simulink model "quadrupedRobot"  (R2020a)
settings: Solver=ode23tb  StartTime=0.0  StopTime=10  RelTol=1e-3
values from neighbouring files (symbols this model uses):
  BodyCenter_To_Arm = BodyLength*0.4    (= 0.24)    [Initial.m]
  BodyLength = 0.6    [Initial.m]
  BodyThick = 0.05    [Initial.m]
  BodyWidth = 0.25    [Initial.m]
  L1 = 0.1*L_total    (= 0.05)    [Initial.m]
  L2 = 0.4*L_total    (= 0.2)    [Initial.m]
  L3 = 0.5*L_total    (= 0.25)    [Initial.m]
  L_total = 0.5    [Initial.m]
  legX = 0.05    [Initial.m]
  legY = 0.05    [Initial.m]
  legZ = 0.05    [Initial.m]
  Mark = 1    [Initial.m]
  X = R_foot*cosd(0:0.2:90)    [Initial.m]
  X_FOOT = ([x_swing x_stance])/1000-S/2/2/1000    [Initial.m]
  Y = R_foot*sind(0:0.2:90)    [Initial.m]
  Y_FOOT = L1    (= 0.05)    [Initial.m]
  Z_FOOT = -L2-L3+Z_trajectory/1000+0.15    [Initial.m]
undefined symbols (not defined in the file or in its folder): Z
libraries: sm_lib x84, nesl_utility x27, Contact_Forces_Lib x5, simulink x1
(part 4 of 4)

== system quadrupedRobot/Robot/RF/upperSys ==
  upperJoint : Inport
  PS-Simulink Converter : nesl_utility/PS-Simulink Converter  PhysicalDomain=network_engine_domain  SubClassName=ps_output  LeftPortType=input  RightPortType=output  PseudoPeriodic=off  Frequencies=[]  Unit=inherit  AffineConversion=off
  R2 : sm_lib/Joints/Revolute Joint  JointMode=Normal  SenseConstraintForce=off  SenseConstraintForceX=off  SenseConstraintForceY=off  SenseConstraintForceZ=off  SenseConstraintTorque=off  SenseConstraintTorqueX=off  SenseConstraintTorqueY=off  SenseConstraintTorqueZ=off  SenseTotalForce=off  SenseTotalForceX=off  SenseTotalForceY=off  SenseTotalForceZ=off  SenseTotalTorque=off  SenseTotalTorqueX=off  SenseTotalTorqueY=off  SenseTotalTorqueZ=off  CompositeWrenchDir=FollowerOnBase  CompositeWrenchFrame=BaseFrame  EquilibriumPosition=0  EquilibriumPositionUnits=deg  SpringStiffness=0  SpringStiffnessUnits=N*m/deg  DampingCoefficient=0  DampingCoefficientUnits=N*m/(deg/s)  TorqueActuationMode=ComputedTorque  MotionActuationMode=InputMotion  SensePosition=off  SenseVelocity=off  SenseAcceleration=off  SenseTorqueForce=on  SenseLowerLimitTorqueForce=off  SenseUpperLimitTorqueForce=off  LowerLimitSpecify=off  LowerLimitBound=-90  LowerLimitBoundUnits=deg  LowerLimitStiffness=1e4  LowerLimitStiffnessUnits=N*m/deg  LowerLimitDamping=10  LowerLimitDampingUnits=N*m/(deg/s)  LowerLimitTransitionRegionWidth=0.1  LowerLimitTransitionRegionWidthUnits=deg  UpperLimitSpecify=off  UpperLimitBound=90  UpperLimitBoundUnits=deg  UpperLimitStiffness=1e4  UpperLimitStiffnessUnits=N*m/deg  UpperLimitDamping=10  UpperLimitDampingUnits=N*m/(deg/s)  UpperLimitTransitionRegionWidth=0.1  UpperLimitTransitionRegionWidthUnits=deg  PositionTargetSpecify=on  PositionTargetPriority=High  PositionTargetValue=0  PositionTargetValueUnits=deg  VelocityTargetSpecify=off  VelocityTargetPriority=High  VelocityTargetValue=0  VelocityTargetValueUnits=deg/s
  Rigid Transform8 : sm_lib/Frames and Transforms/Rigid Transform  TranslationMethod=None  TranslationStandardOffset=0  TranslationLengthUnit=m  TranslationStandardAxis=+Z  TranslationCartesianOffset=[0 0 0]  TranslationROffset=0  TranslationROffsetUnits=m  TranslationZOffset=0  TranslationZOffsetUnits=m  TranslationThetaOffset=0  TranslationThetaOffsetUnits=deg  RotationMethod=StandardAxis  RotationAngleUnits=deg  RotationStandardAxis=+X  RotationAngle=90  RotationArbitraryAxis=[0 0 1]  FollAlignAxisA=+X  BaseAlignAxisA=+Y  FollAlignAxisB=+Y  BaseAlignAxisB=+Z  RotationSequenceAxes=FollowerAxes  RotationSequence=XYX  RotationSequenceAngles=[0 0 0]  RotationSequenceAnglesUnits=deg  RotationMatrix=[1 0 0; 0 1 0; 0 0 1]
  Rigid Transform9 : sm_lib/Frames and Transforms/Rigid Transform  TranslationMethod=None  TranslationStandardOffset=0  TranslationLengthUnit=m  TranslationStandardAxis=+Z  TranslationCartesianOffset=[0 0 0]  TranslationROffset=0  TranslationROffsetUnits=m  TranslationZOffset=0  TranslationZOffsetUnits=m  TranslationThetaOffset=0  TranslationThetaOffsetUnits=deg  RotationMethod=StandardAxis  RotationAngleUnits=deg  RotationStandardAxis=+X  RotationAngle=90  RotationArbitraryAxis=[0 0 1]  FollAlignAxisA=+X  BaseAlignAxisA=+Y  FollAlignAxisB=+Y  BaseAlignAxisB=+Z  RotationSequenceAxes=FollowerAxes  RotationSequence=XYX  RotationSequenceAngles=[0 0 0]  RotationSequenceAnglesUnits=deg  RotationMatrix=[1 0 0; 0 1 0; 0 0 1]
  Simulink-PS Converter4 : nesl_utility/Simulink-PS Converter  PhysicalDomain=network_engine_domain  SubClassName=ps_input  LeftPortType=input  RightPortType=output  PseudoPeriodic=off  Frequencies=[]  NoiseDistribution=none  NoiseParameters=[]  Unit=1  AffineConversion=off  FilteringAndDerivatives=filter  SimscapeFilterOrder=2  InputFilterTimeConstant=0.001  UdotUserProvided=0
  B1 : PMIOPort  Side=Left
  B2 : PMIOPort  Port=2  Side=Right
  Torque : Outport
  wires:
  upperJoint/1 -> Simulink-PS Converter4/1
  PS-Simulink Converter/1 -> Torque/1
  connections:
  Rigid Transform9/LConn1 -- B2/RConn1
  Rigid Transform8/LConn1 -- B1/RConn1
  R2/RConn1 -- Rigid Transform9/RConn1
  Rigid Transform8/RConn1 -- R2/LConn1
  Simulink-PS Converter4/RConn1 -- R2/LConn2
  PS-Simulink Converter/LConn1 -- R2/RConn2

== system quadrupedRobot/Robot/RR/Subsystem ==
  shoulderJoint : Inport
  R1 : sm_lib/Joints/Revolute Joint  JointMode=Normal  SenseConstraintForce=off  SenseConstraintForceX=off  SenseConstraintForceY=off  SenseConstraintForceZ=off  SenseConstraintTorque=off  SenseConstraintTorqueX=off  SenseConstraintTorqueY=off  SenseConstraintTorqueZ=off  SenseTotalForce=off  SenseTotalForceX=off  SenseTotalForceY=off  SenseTotalForceZ=off  SenseTotalTorque=off  SenseTotalTorqueX=off  SenseTotalTorqueY=off  SenseTotalTorqueZ=off  CompositeWrenchDir=FollowerOnBase  CompositeWrenchFrame=BaseFrame  EquilibriumPosition=0  EquilibriumPositionUnits=deg  SpringStiffness=0  SpringStiffnessUnits=N*m/deg  DampingCoefficient=0  DampingCoefficientUnits=N*m/(deg/s)  TorqueActuationMode=ComputedTorque  MotionActuationMode=InputMotion  SensePosition=off  SenseVelocity=off  SenseAcceleration=off  SenseTorqueForce=off  SenseLowerLimitTorqueForce=off  SenseUpperLimitTorqueForce=off  LowerLimitSpecify=off  LowerLimitBound=-90  LowerLimitBoundUnits=deg  LowerLimitStiffness=1e4  LowerLimitStiffnessUnits=N*m/deg  LowerLimitDamping=10  LowerLimitDampingUnits=N*m/(deg/s)  LowerLimitTransitionRegionWidth=0.1  LowerLimitTransitionRegionWidthUnits=deg  UpperLimitSpecify=off  UpperLimitBound=90  UpperLimitBoundUnits=deg  UpperLimitStiffness=1e4  UpperLimitStiffnessUnits=N*m/deg  UpperLimitDamping=10  UpperLimitDampingUnits=N*m/(deg/s)  UpperLimitTransitionRegionWidth=0.1  UpperLimitTransitionRegionWidthUnits=deg  PositionTargetSpecify=on  PositionTargetPriority=High  PositionTargetValue=0  PositionTargetValueUnits=deg  VelocityTargetSpecify=off  VelocityTargetPriority=High  VelocityTargetValue=0  VelocityTargetValueUnits=deg/s
  Rigid Transform8 : sm_lib/Frames and Transforms/Rigid Transform  TranslationMethod=None  TranslationStandardOffset=0  TranslationLengthUnit=m  TranslationStandardAxis=+Z  TranslationCartesianOffset=[0 0 0]  TranslationROffset=0  TranslationROffsetUnits=m  TranslationZOffset=0  TranslationZOffsetUnits=m  TranslationThetaOffset=0  TranslationThetaOffsetUnits=deg  RotationMethod=StandardAxis  RotationAngleUnits=deg  RotationStandardAxis=+Y  RotationAngle=90  RotationArbitraryAxis=[0 0 1]  FollAlignAxisA=+X  BaseAlignAxisA=+Y  FollAlignAxisB=+Y  BaseAlignAxisB=+Z  RotationSequenceAxes=FollowerAxes  RotationSequence=XYX  RotationSequenceAngles=[0 0 0]  RotationSequenceAnglesUnits=deg  RotationMatrix=[1 0 0; 0 1 0; 0 0 1]
  Rigid Transform9 : sm_lib/Frames and Transforms/Rigid Transform  TranslationMethod=None  TranslationStandardOffset=0  TranslationLengthUnit=m  TranslationStandardAxis=+Z  TranslationCartesianOffset=[0 0 0]  TranslationROffset=0  TranslationROffsetUnits=m  TranslationZOffset=0  TranslationZOffsetUnits=m  TranslationThetaOffset=0  TranslationThetaOffsetUnits=deg  RotationMethod=StandardAxis  RotationAngleUnits=deg  RotationStandardAxis=+Y  RotationAngle=90  RotationArbitraryAxis=[0 0 1]  FollAlignAxisA=+X  BaseAlignAxisA=+Y  FollAlignAxisB=+Y  BaseAlignAxisB=+Z  RotationSequenceAxes=FollowerAxes  RotationSequence=XYX  RotationSequenceAngles=[0 0 0]  RotationSequenceAnglesUnits=deg  RotationMatrix=[1 0 0; 0 1 0; 0 0 1]
  Simulink-PS Converter4 : nesl_utility/Simulink-PS Converter  PhysicalDomain=network_engine_domain  SubClassName=ps_input  LeftPortType=input  RightPortType=output  PseudoPeriodic=off  Frequencies=[]  NoiseDistribution=none  NoiseParameters=[]  Unit=1  AffineConversion=off  FilteringAndDerivatives=filter  SimscapeFilterOrder=2  InputFilterTimeConstant=0.001  UdotUserProvided=0
  B1 : PMIOPort  Side=Left
  B2 : PMIOPort  Port=2  Side=Right
  wires:
  shoulderJoint/1 -> Simulink-PS Converter4/1
  connections:
  Rigid Transform8/RConn1 -- R1/LConn1
  Simulink-PS Converter4/RConn1 -- R1/LConn2
  R1/RConn1 -- Rigid Transform9/RConn1
  Rigid Transform8/LConn1 -- B1/RConn1
  Rigid Transform9/LConn1 -- B2/RConn1

== system quadrupedRobot/Robot/RR/Subsystem1 ==
  upperJoint : Inport
  R2 : sm_lib/Joints/Revolute Joint  JointMode=Normal  SenseConstraintForce=off  SenseConstraintForceX=off  SenseConstraintForceY=off  SenseConstraintForceZ=off  SenseConstraintTorque=off  SenseConstraintTorqueX=off  SenseConstraintTorqueY=off  SenseConstraintTorqueZ=off  SenseTotalForce=off  SenseTotalForceX=off  SenseTotalForceY=off  SenseTotalForceZ=off  SenseTotalTorque=off  SenseTotalTorqueX=off  SenseTotalTorqueY=off  SenseTotalTorqueZ=off  CompositeWrenchDir=FollowerOnBase  CompositeWrenchFrame=BaseFrame  EquilibriumPosition=0  EquilibriumPositionUnits=deg  SpringStiffness=0  SpringStiffnessUnits=N*m/deg  DampingCoefficient=0  DampingCoefficientUnits=N*m/(deg/s)  TorqueActuationMode=ComputedTorque  MotionActuationMode=InputMotion  SensePosition=off  SenseVelocity=off  SenseAcceleration=off  SenseTorqueForce=off  SenseLowerLimitTorqueForce=off  SenseUpperLimitTorqueForce=off  LowerLimitSpecify=off  LowerLimitBound=-90  LowerLimitBoundUnits=deg  LowerLimitStiffness=1e4  LowerLimitStiffnessUnits=N*m/deg  LowerLimitDamping=10  LowerLimitDampingUnits=N*m/(deg/s)  LowerLimitTransitionRegionWidth=0.1  LowerLimitTransitionRegionWidthUnits=deg  UpperLimitSpecify=off  UpperLimitBound=90  UpperLimitBoundUnits=deg  UpperLimitStiffness=1e4  UpperLimitStiffnessUnits=N*m/deg  UpperLimitDamping=10  UpperLimitDampingUnits=N*m/(deg/s)  UpperLimitTransitionRegionWidth=0.1  UpperLimitTransitionRegionWidthUnits=deg  PositionTargetSpecify=on  PositionTargetPriority=High  PositionTargetValue=0  PositionTargetValueUnits=deg  VelocityTargetSpecify=off  VelocityTargetPriority=High  VelocityTargetValue=0  VelocityTargetValueUnits=deg/s
  Rigid Transform8 : sm_lib/Frames and Transforms/Rigid Transform  TranslationMethod=None  TranslationStandardOffset=0  TranslationLengthUnit=m  TranslationStandardAxis=+Z  TranslationCartesianOffset=[0 0 0]  TranslationROffset=0  TranslationROffsetUnits=m  TranslationZOffset=0  TranslationZOffsetUnits=m  TranslationThetaOffset=0  TranslationThetaOffsetUnits=deg  RotationMethod=StandardAxis  RotationAngleUnits=deg  RotationStandardAxis=+X  RotationAngle=90  RotationArbitraryAxis=[0 0 1]  FollAlignAxisA=+X  BaseAlignAxisA=+Y  FollAlignAxisB=+Y  BaseAlignAxisB=+Z  RotationSequenceAxes=FollowerAxes  RotationSequence=XYX  RotationSequenceAngles=[0 0 0]  RotationSequenceAnglesUnits=deg  RotationMatrix=[1 0 0; 0 1 0; 0 0 1]
  Rigid Transform9 : sm_lib/Frames and Transforms/Rigid Transform  TranslationMethod=None  TranslationStandardOffset=0  TranslationLengthUnit=m  TranslationStandardAxis=+Z  TranslationCartesianOffset=[0 0 0]  TranslationROffset=0  TranslationROffsetUnits=m  TranslationZOffset=0  TranslationZOffsetUnits=m  TranslationThetaOffset=0  TranslationThetaOffsetUnits=deg  RotationMethod=StandardAxis  RotationAngleUnits=deg  RotationStandardAxis=+X  RotationAngle=90  RotationArbitraryAxis=[0 0 1]  FollAlignAxisA=+X  BaseAlignAxisA=+Y  FollAlignAxisB=+Y  BaseAlignAxisB=+Z  RotationSequenceAxes=FollowerAxes  RotationSequence=XYX  RotationSequenceAngles=[0 0 0]  RotationSequenceAnglesUnits=deg  RotationMatrix=[1 0 0; 0 1 0; 0 0 1]
  Simulink-PS Converter4 : nesl_utility/Simulink-PS Converter  PhysicalDomain=network_engine_domain  SubClassName=ps_input  LeftPortType=input  RightPortType=output  PseudoPeriodic=off  Frequencies=[]  NoiseDistribution=none  NoiseParameters=[]  Unit=1  AffineConversion=off  FilteringAndDerivatives=filter  SimscapeFilterOrder=2  InputFilterTimeConstant=0.001  UdotUserProvided=0
  B1 : PMIOPort  Side=Left
  B2 : PMIOPort  Port=2  Side=Right
  wires:
  upperJoint/1 -> Simulink-PS Converter4/1
  connections:
  Rigid Transform9/LConn1 -- B2/RConn1
  Rigid Transform8/LConn1 -- B1/RConn1
  R2/RConn1 -- Rigid Transform9/RConn1
  Rigid Transform8/RConn1 -- R2/LConn1
  Simulink-PS Converter4/RConn1 -- R2/LConn2

== system quadrupedRobot/Robot/RR/Subsystem2 ==
  lowerJoint : Inport
  R3 : sm_lib/Joints/Revolute Joint  JointMode=Normal  SenseConstraintForce=off  SenseConstraintForceX=off  SenseConstraintForceY=off  SenseConstraintForceZ=off  SenseConstraintTorque=off  SenseConstraintTorqueX=off  SenseConstraintTorqueY=off  SenseConstraintTorqueZ=off  SenseTotalForce=off  SenseTotalForceX=off  SenseTotalForceY=off  SenseTotalForceZ=off  SenseTotalTorque=off  SenseTotalTorqueX=off  SenseTotalTorqueY=off  SenseTotalTorqueZ=off  CompositeWrenchDir=FollowerOnBase  CompositeWrenchFrame=BaseFrame  EquilibriumPosition=0  EquilibriumPositionUnits=deg  SpringStiffness=0  SpringStiffnessUnits=N*m/deg  DampingCoefficient=0  DampingCoefficientUnits=N*m/(deg/s)  TorqueActuationMode=ComputedTorque  MotionActuationMode=InputMotion  SensePosition=off  SenseVelocity=off  SenseAcceleration=off  SenseTorqueForce=off  SenseLowerLimitTorqueForce=off  SenseUpperLimitTorqueForce=off  LowerLimitSpecify=off  LowerLimitBound=-90  LowerLimitBoundUnits=deg  LowerLimitStiffness=1e4  LowerLimitStiffnessUnits=N*m/deg  LowerLimitDamping=10  LowerLimitDampingUnits=N*m/(deg/s)  LowerLimitTransitionRegionWidth=0.1  LowerLimitTransitionRegionWidthUnits=deg  UpperLimitSpecify=off  UpperLimitBound=90  UpperLimitBoundUnits=deg  UpperLimitStiffness=1e4  UpperLimitStiffnessUnits=N*m/deg  UpperLimitDamping=10  UpperLimitDampingUnits=N*m/(deg/s)  UpperLimitTransitionRegionWidth=0.1  UpperLimitTransitionRegionWidthUnits=deg  PositionTargetSpecify=on  PositionTargetPriority=High  PositionTargetValue=0  PositionTargetValueUnits=deg  VelocityTargetSpecify=off  VelocityTargetPriority=High  VelocityTargetValue=0  VelocityTargetValueUnits=deg/s
  Rigid Transform8 : sm_lib/Frames and Transforms/Rigid Transform  TranslationMethod=None  TranslationStandardOffset=0  TranslationLengthUnit=m  TranslationStandardAxis=+Z  TranslationCartesianOffset=[0 0 0]  TranslationROffset=0  TranslationROffsetUnits=m  TranslationZOffset=0  TranslationZOffsetUnits=m  TranslationThetaOffset=0  TranslationThetaOffsetUnits=deg  RotationMethod=StandardAxis  RotationAngleUnits=deg  RotationStandardAxis=+X  RotationAngle=90  RotationArbitraryAxis=[0 0 1]  FollAlignAxisA=+X  BaseAlignAxisA=+Y  FollAlignAxisB=+Y  BaseAlignAxisB=+Z  RotationSequenceAxes=FollowerAxes  RotationSequence=XYX  RotationSequenceAngles=[0 0 0]  RotationSequenceAnglesUnits=deg  RotationMatrix=[1 0 0; 0 1 0; 0 0 1]
  Rigid Transform9 : sm_lib/Frames and Transforms/Rigid Transform  TranslationMethod=None  TranslationStandardOffset=0  TranslationLengthUnit=m  TranslationStandardAxis=+Z  TranslationCartesianOffset=[0 0 0]  TranslationROffset=0  TranslationROffsetUnits=m  TranslationZOffset=0  TranslationZOffsetUnits=m  TranslationThetaOffset=0  TranslationThetaOffsetUnits=deg  RotationMethod=StandardAxis  RotationAngleUnits=deg  RotationStandardAxis=+X  RotationAngle=90  RotationArbitraryAxis=[0 0 1]  FollAlignAxisA=+X  BaseAlignAxisA=+Y  FollAlignAxisB=+Y  BaseAlignAxisB=+Z  RotationSequenceAxes=FollowerAxes  RotationSequence=XYX  RotationSequenceAngles=[0 0 0]  RotationSequenceAnglesUnits=deg  RotationMatrix=[1 0 0; 0 1 0; 0 0 1]
  Simulink-PS Converter : nesl_utility/Simulink-PS Converter  PhysicalDomain=network_engine_domain  SubClassName=ps_input  LeftPortType=input  RightPortType=output  PseudoPeriodic=off  Frequencies=[]  NoiseDistribution=none  NoiseParameters=[]  Unit=1  AffineConversion=off  FilteringAndDerivatives=filter  SimscapeFilterOrder=2  InputFilterTimeConstant=0.001  UdotUserProvided=0
  B1 : PMIOPort  Side=Left
  B2 : PMIOPort  Port=2  Side=Right
  wires:
  lowerJoint/1 -> Simulink-PS Converter/1
  connections:
  Rigid Transform9/LConn1 -- B2/RConn1
  Rigid Transform8/LConn1 -- B1/RConn1
  R3/RConn1 -- Rigid Transform9/RConn1
  Simulink-PS Converter/RConn1 -- R3/LConn2
  Rigid Transform8/RConn1 -- R3/LConn1

== system quadrupedRobot/controller/原地机身ROLL PITCH YAW三角变化演示（正确）/LF_CONTROL ==
  Theta123 : Inport
  Demux : Demux  Outputs=3
  Gain : Gain  Gain=-1
  ToRad : Gain  Gain=pi/180
  tag scope: LF_lower=global, LF_shoulder=global, LF_upper=global
  wires:
  Theta123/1 -> ToRad/1
  Demux/3 -> [LF_lower]
  Demux/1 -> Gain/1
  Demux/2 -> [LF_upper]
  ToRad/1 -> Demux/1
  Gain/1 -> [LF_shoulder]

== system quadrupedRobot/controller/原地机身ROLL PITCH YAW三角变化演示（正确）/LR_CONTROL ==
  Theta123 : Inport
  Demux : Demux  Outputs=3
  Gain : Gain  Gain=-1
  ToRad : Gain  Gain=pi/180
  tag scope: LR_lower=global, LR_shoulder=global, LR_upper=global
  wires:
  Theta123/1 -> ToRad/1
  Demux/3 -> [LR_lower]
  Demux/1 -> Gain/1
  Demux/2 -> [LR_upper]
  ToRad/1 -> Demux/1
  Gain/1 -> [LR_shoulder]

== system quadrupedRobot/controller/原地机身ROLL PITCH YAW三角变化演示（正确）/RF_CONTROL ==
  Theta123 : Inport
  Demux : Demux  Outputs=3
  ToRad : Gain  Gain=pi/180
  tag scope: RF_lower=global, RF_shoulder=global, RF_upper=global
  wires:
  Demux/1 -> [RF_shoulder]
  Demux/3 -> [RF_lower]
  Demux/2 -> [RF_upper]
  Theta123/1 -> ToRad/1
  ToRad/1 -> Demux/1

== system quadrupedRobot/controller/原地机身ROLL PITCH YAW三角变化演示（正确）/RR_CONTROL ==
  Theta123 : Inport
  Demux : Demux  Outputs=3
  ToRad : Gain  Gain=pi/180
  tag scope: RR_lower=global, RR_shoulder=global, RR_upper=global
  wires:
  Theta123/1 -> ToRad/1
  Demux/3 -> [RR_lower]
  Demux/1 -> [RR_shoulder]
  Demux/2 -> [RR_upper]
  ToRad/1 -> Demux/1

== system quadrupedRobot/controller/原地机身ROLL PITCH YAW三角变化演示（正确）/初始位置发生器（每条腿相同） ==
  Init_X : Constant  Value=X_FOOT(1)
  Init_Y : Constant  Value=Y_FOOT(1)
  Init_Z : Constant  Value=Z_FOOT(1)
  Init_x : Outport
  Init_y : Outport  Port=2
  Init_z : Outport  Port=3
  wires:
  Init_X/1 -> Init_x/1
  Init_Y/1 -> Init_y/1
  Init_Z/1 -> Init_z/1

== system quadrupedRobot/controller/原地机身ROLL角变化演示/LF_CONTROL ==
  Theta123 : Inport
  Demux : Demux  Outputs=3
  Gain : Gain  Gain=-1
  ToRad : Gain  Gain=pi/180
  tag scope: LF_lower=global, LF_shoulder=global, LF_upper=global
  wires:
  Theta123/1 -> ToRad/1
  Demux/3 -> [LF_lower]
  Demux/1 -> Gain/1
  Demux/2 -> [LF_upper]
  ToRad/1 -> Demux/1
  Gain/1 -> [LF_shoulder]

== system quadrupedRobot/controller/原地机身ROLL角变化演示/LR_CONTROL ==
  Theta123 : Inport
  Demux : Demux  Outputs=3
  Gain : Gain  Gain=-1
  ToRad : Gain  Gain=pi/180
  tag scope: LR_lower=global, LR_shoulder=global, LR_upper=global
  wires:
  Theta123/1 -> ToRad/1
  Demux/3 -> [LR_lower]
  Demux/1 -> Gain/1
  Demux/2 -> [LR_upper]
  ToRad/1 -> Demux/1
  Gain/1 -> [LR_shoulder]

== system quadrupedRobot/controller/原地机身ROLL角变化演示/RF_CONTROL ==
  Theta123 : Inport
  Demux : Demux  Outputs=3
  ToRad : Gain  Gain=pi/180
  tag scope: RF_lower=global, RF_shoulder=global, RF_upper=global
  wires:
  Demux/1 -> [RF_shoulder]
  Demux/3 -> [RF_lower]
  Demux/2 -> [RF_upper]
  Theta123/1 -> ToRad/1
  ToRad/1 -> Demux/1

== system quadrupedRobot/controller/原地机身ROLL角变化演示/RR_CONTROL ==
  Theta123 : Inport
  Demux : Demux  Outputs=3
  ToRad : Gain  Gain=pi/180
  tag scope: RR_lower=global, RR_shoulder=global, RR_upper=global
  wires:
  Theta123/1 -> ToRad/1
  Demux/3 -> [RR_lower]
  Demux/1 -> [RR_shoulder]
  Demux/2 -> [RR_upper]
  ToRad/1 -> Demux/1

== system quadrupedRobot/controller/原地机身ROLL角变化演示/初始位置发生器（每条腿相同） ==
  Init_X : Constant  Value=X_FOOT(1)
  Init_Y : Constant  Value=L1
  Init_Z : Constant  Value=Z_FOOT(1)
  Init_x : Outport
  Init_y : Outport  Port=2
  Init_z : Outport  Port=3
  wires:
  Init_X/1 -> Init_x/1
  Init_Y/1 -> Init_y/1
  Init_Z/1 -> Init_z/1

== system quadrupedRobot/controller/原地机身YAW角变化演示（有误）/LF_CONTROL ==
  Theta123 : Inport
  Demux : Demux  Outputs=3
  Gain : Gain  Gain=-1
  ToRad : Gain  Gain=pi/180
  tag scope: LF_lower=global, LF_shoulder=global, LF_upper=global
  wires:
  Gain/1 -> [LF_shoulder]
  ToRad/1 -> Demux/1
  Demux/2 -> [LF_upper]
  Demux/1 -> Gain/1
  Demux/3 -> [LF_lower]
  Theta123/1 -> ToRad/1

== system quadrupedRobot/controller/原地机身YAW角变化演示（有误）/LR_CONTROL ==
  Theta123 : Inport
  Demux : Demux  Outputs=3
  Gain : Gain  Gain=-1
  ToRad : Gain  Gain=pi/180
  tag scope: LR_lower=global, LR_shoulder=global, LR_upper=global
  wires:
  Gain/1 -> [LR_shoulder]
  ToRad/1 -> Demux/1
  Demux/2 -> [LR_upper]
  Demux/1 -> Gain/1
  Demux/3 -> [LR_lower]
  Theta123/1 -> ToRad/1

== system quadrupedRobot/controller/原地机身YAW角变化演示（有误）/RF_CONTROL ==
  Theta123 : Inport
  Demux : Demux  Outputs=3
  ToRad : Gain  Gain=pi/180
  tag scope: RF_lower=global, RF_shoulder=global, RF_upper=global
  wires:
  ToRad/1 -> Demux/1
  Theta123/1 -> ToRad/1
  Demux/2 -> [RF_upper]
  Demux/3 -> [RF_lower]
  Demux/1 -> [RF_shoulder]

== system quadrupedRobot/controller/原地机身YAW角变化演示（有误）/RR_CONTROL ==
  Theta123 : Inport
  Demux : Demux  Outputs=3
  ToRad : Gain  Gain=pi/180
  tag scope: RR_lower=global, RR_shoulder=global, RR_upper=global
  wires:
  ToRad/1 -> Demux/1
  Demux/2 -> [RR_upper]
  Demux/1 -> [RR_shoulder]
  Demux/3 -> [RR_lower]
  Theta123/1 -> ToRad/1

== system quadrupedRobot/controller/原地机身YAW角变化演示（有误）/初始位置发生器（每条腿相同） ==
  Init_X : Constant  Value=X_FOOT(1)
  Init_Y : Constant  Value=Y_FOOT(1)
  Init_Z : Constant  Value=Z_FOOT(1)
  Init_x : Outport
  Init_y : Outport  Port=2
  Init_z : Outport  Port=3
  wires:
  Init_Z/1 -> Init_z/1
  Init_Y/1 -> Init_y/1
  Init_X/1 -> Init_x/1

== system quadrupedRobot/controller/对角步态演示/LF_CONTROL ==
  Theta123 : Inport
  Demux : Demux  Outputs=3
  Gain : Gain  Gain=-1
  ToRad : Gain  Gain=pi/180
  tag scope: LF_lower=global, LF_shoulder=global, LF_upper=global
  wires:
  Theta123/1 -> ToRad/1
  Demux/3 -> [LF_lower]
  Demux/1 -> Gain/1
  Demux/2 -> [LF_upper]
  ToRad/1 -> Demux/1
  Gain/1 -> [LF_shoulder]

== system quadrupedRobot/controller/对角步态演示/LR_CONTROL ==
  Theta123 : Inport
  Demux : Demux  Outputs=3
  Gain : Gain  Gain=-1
  ToRad : Gain  Gain=pi/180
  tag scope: LR_lower=global, LR_shoulder=global, LR_upper=global
  wires:
  Theta123/1 -> ToRad/1
  Demux/3 -> [LR_lower]
  Demux/1 -> Gain/1
  Demux/2 -> [LR_upper]
  ToRad/1 -> Demux/1
  Gain/1 -> [LR_shoulder]

== system quadrupedRobot/controller/对角步态演示/RF_CONTROL ==
  Theta123 : Inport
  Demux : Demux  Outputs=3
  ToRad : Gain  Gain=pi/180
  tag scope: RF_lower=global, RF_shoulder=global, RF_upper=global
  wires:
  Demux/1 -> [RF_shoulder]
  Demux/3 -> [RF_lower]
  Demux/2 -> [RF_upper]
  Theta123/1 -> ToRad/1
  ToRad/1 -> Demux/1

== system quadrupedRobot/controller/对角步态演示/RR_CONTROL ==
  Theta123 : Inport
  Demux : Demux  Outputs=3
  ToRad : Gain  Gain=pi/180
  tag scope: RR_lower=global, RR_shoulder=global, RR_upper=global
  wires:
  Theta123/1 -> ToRad/1
  Demux/3 -> [RR_lower]
  Demux/1 -> [RR_shoulder]
  Demux/2 -> [RR_upper]
  ToRad/1 -> Demux/1

== system quadrupedRobot/controller/对角步态演示/初始位置发生器（每条腿相同） ==
  Init_X : Constant  Value=X_FOOT(1)
  Init_Y : Constant  Value=Y_FOOT(1)
  Init_Z : Constant  Value=Z_FOOT(1)
  Init_x : Outport
  Init_y : Outport  Port=2
  Init_z : Outport  Port=3
  wires:
  Init_X/1 -> Init_x/1
  Init_Y/1 -> Init_y/1
  Init_Z/1 -> Init_z/1

== system quadrupedRobot/controller/对角步态演示/对角步态坐标生成器 ==
  Constant1 : Constant
  Counter Limited2 : simulink/Sources/Counter Limited  uplimit=length(Z_FOOT)-1  tsamp=0.0001
  Sum2 : Sum  Inputs=|++
  X1 : Lookup_n-D  NumberOfTableDimensions=1  BreakpointsForDimension1=[1:length(Z_FOOT)]  Table=X_FOOT  InternalRulePriority=Speed  RndMeth=Simplest  InputSameDT=on
  X2 : Lookup_n-D  NumberOfTableDimensions=1  BreakpointsForDimension1=[1:length(Z_FOOT)]  Table="[X_FOOT(length(x_swing)+1:end)  X_FOOT(1:length(x_swing))]"  InternalRulePriority=Speed  RndMeth=Simplest  InputSameDT=on
  Y : Constant  Value=L1
  Z1 : Lookup_n-D  NumberOfTableDimensions=1  BreakpointsForDimension1=[1:length(Z_FOOT)]  Table=Z_FOOT  InternalRulePriority=Speed  RndMeth=Simplest  InputSameDT=on
  Z2 : Lookup_n-D  NumberOfTableDimensions=1  BreakpointsForDimension1=[1:length(Z_FOOT)]  Table=[Z_FOOT(length(x_swing)+1:end) Z_FOOT(1:length(x_swing))]  InternalRulePriority=Speed  RndMeth=Simplest  InputSameDT=on
  延时为了与Chart一致 : Delay  DelayLength=3000
  x2 : Outport
  z2 : Outport  Port=2
  x1 : Outport  Port=3
  z1 : Outport  Port=4
  y : Outport  Port=5
  wires:
  延时为了与Chart一致/1 -> Z1/1, X1/1, Z2/1, X2/1
  Z2/1 -> z2/1
  Counter Limited2/1 -> Sum2/1
  X2/1 -> x2/1
  Z1/1 -> z1/1
  Y/1 -> y/1
  Sum2/1 -> 延时为了与Chart一致/1
  Constant1/1 -> Sum2/2
  X1/1 -> x1/1

== matlab function quadrupedRobot/controller/原地机身ROLL角变化演示/Kinematics3 ==
  data: POrAngle_RF output; XYZ input; POrAngle_RR output; POrAngle_LF output; POrAngle_LR output; L1 parameter; L2 parameter; L3 parameter; Mark parameter
function [POrAngle_RF,POrAngle_RR,POrAngle_LF,POrAngle_LR] = fcn(XYZ, L1, L2, L3, Mark)%L1 L2 L3 MARK是内置数值
    



%     RF_XYZ = XYZ(1:3);%右前腿坐标
%     RR_XYZ = XYZ(4:6);
%     LF_XYZ = XYZ(7:9);
%     LR_XYZ = XYZ(10:12);
    
   POrAngle_RF = zeros(1,3);
   POrAngle_RR = zeros(1,3);
   POrAngle_LF = zeros(1,3);
   POrAngle_LR = zeros(1,3);
%     POrAngle1=0;
%     POrAngle2=0;
%     POrAngle3=0;
    Theta_Total = zeros(4,3);%用以装载角度
    XYZ_Total   = zeros(4,3);%用以装载XYZ
    switch Mark
        case 1 %计算逆运动学
           for K=1:4  %依次算四条腿的逆解
                [POrAngle1,POrAngle2,POrAngle3]=inverseKinematics(L1,L2,L3,XYZ(3*K-2),XYZ(3*K-1),XYZ(3*K));
                Theta_Total(K,1) = POrAngle1;
                Theta_Total(K,2) = POrAngle2;
                Theta_Total(K,3) = POrAngle3;
           end
           POrAngle_RF = Theta_Total(1,:) ;
           POrAngle_RR = Theta_Total(2,:) ;
           POrAngle_LF = Theta_Total(3,:) ;
           POrAngle_LR = Theta_Total(4,:) ;
        case 0 
            for K=1:4  %依次算四条腿的逆解
                [POrAngle1,POrAngle2,POrAngle3]=forwardKinematics(L1,L2,L3,XYZ(3*K-2),XYZ(3*K-1),XYZ(3*K));
                XYZ_Total(K,1) = POrAngle1;
                XYZ_Total(K,2) = POrAngle2;
                XYZ_Total(K,3) = POrAngle3;
           end
           POrAngle_RF = XYZ_Total(1,:) ;
           POrAngle_RR = XYZ_Total(2,:) ;
           POrAngle_LF = XYZ_Total(3,:) ;
           POrAngle_LR = XYZ_Total(4,:) ;
    end
    
    
    
    
    
    
    
    
   
    
end



function [x,y,z]=forwardKinematics(a,L1,L2,theta0,theta1,theta2)
    
    H = L1*cosd(theta1)+L2*cosd(theta1+theta2);
    x = L1*sind(theta1)+L2*sind(theta1+theta2);
    z = -H*cosd(theta0)+a*sind(theta0);
    y = a*cosd(theta0)+H*sind(theta0);
end

function [theta0,theta1,theta2]=inverseKinematics(a,L1,L2,x,y,z)

    h = a;
    hu = L1;
    hl = L2;
    %
    y = -y;
    z = -(abs(z));
    dyz = sqrt(y^2+z^2);
    lyz = sqrt(dyz^2-a^2);
    gamma_yz = -atand(y/z);
    gamma_h_offset = -atand(h/lyz);
    gamma = gamma_yz-gamma_h_offset;
    theta0 = -gamma;
    %
    lxzp =  sqrt(lyz^2+x^2);
    n = (lxzp^2-hl^2-hu^2)/2/hu;
    beta = -acosd(n/hl);
    theta2 = -beta ;
    %
    alfa_xzp = -atand(x/lyz);
    alfa_off = acosd((hu+n)/lxzp);
    alfa = alfa_xzp+alfa_off;
    theta1 = -alfa;

end

== matlab function quadrupedRobot/controller/原地机身YAW角变化演示（有误）/Kinematics ==
  data: POrAngle_RF output; XYZ input; POrAngle_RR output; POrAngle_LF output; POrAngle_LR output; L1 parameter; L2 parameter; L3 parameter; Mark parameter
function [POrAngle_RF,POrAngle_RR,POrAngle_LF,POrAngle_LR] = fcn(XYZ, L1, L2, L3, Mark)%L1 L2 L3 MARK是内置数值
    



%     RF_XYZ = XYZ(1:3);%右前腿坐标
%     RR_XYZ = XYZ(4:6);
%     LF_XYZ = XYZ(7:9);
%     LR_XYZ = XYZ(10:12);
    
   POrAngle_RF = zeros(1,3);
   POrAngle_RR = zeros(1,3);
   POrAngle_LF = zeros(1,3);
   POrAngle_LR = zeros(1,3);
%     POrAngle1=0;
%     POrAngle2=0;
%     POrAngle3=0;
    Theta_Total = zeros(4,3);%用以装载角度
    XYZ_Total   = zeros(4,3);%用以装载XYZ
    switch Mark
        case 1 %计算逆运动学
           for K=1:4  %依次算四条腿的逆解
                [POrAngle1,POrAngle2,POrAngle3]=inverseKinematics(L1,L2,L3,XYZ(3*K-2),XYZ(3*K-1),XYZ(3*K));
                Theta_Total(K,1) = POrAngle1;
                Theta_Total(K,2) = POrAngle2;
                Theta_Total(K,3) = POrAngle3;
           end
           POrAngle_RF = Theta_Total(1,:) ;
           POrAngle_RR = Theta_Total(2,:) ;
           POrAngle_LF = Theta_Total(3,:) ;
           POrAngle_LR = Theta_Total(4,:) ;
        case 0 
            for K=1:4  %依次算四条腿的逆解
                [POrAngle1,POrAngle2,POrAngle3]=forwardKinematics(L1,L2,L3,XYZ(3*K-2),XYZ(3*K-1),XYZ(3*K));
                XYZ_Total(K,1) = POrAngle1;
                XYZ_Total(K,2) = POrAngle2;
                XYZ_Total(K,3) = POrAngle3;
           end
           POrAngle_RF = XYZ_Total(1,:) ;
           POrAngle_RR = XYZ_Total(2,:) ;
           POrAngle_LF = XYZ_Total(3,:) ;
           POrAngle_LR = XYZ_Total(4,:) ;
    end
    
    
    
    
    
    
    
    
   
    
end



function [x,y,z]=forwardKinematics(a,L1,L2,theta0,theta1,theta2)
    
    H = L1*cosd(theta1)+L2*cosd(theta1+theta2);
    x = L1*sind(theta1)+L2*sind(theta1+theta2);
    z = -H*cosd(theta0)+a*sind(theta0);
    y = a*cosd(theta0)+H*sind(theta0);
end

function [theta0,theta1,theta2]=inverseKinematics(a,L1,L2,x,y,z)

    h = a;
    hu = L1;
    hl = L2;
    %
    y = -y;
    z = -(abs(z));
    dyz = sqrt(y^2+z^2);
    lyz = sqrt(dyz^2-a^2);
    gamma_yz = -atand(y/z);
    gamma_h_offset = -atand(h/lyz);
    gamma = gamma_yz-gamma_h_offset;
    theta0 = -gamma;
    %
    lxzp =  sqrt(lyz^2+x^2);
    n = (lxzp^2-hl^2-hu^2)/2/hu;
    beta = -acosd(n/hl);
    theta2 = -beta ;
    %
    alfa_xzp = -atand(x/lyz);
    alfa_off = acosd((hu+n)/lxzp);
    alfa = alfa_xzp+alfa_off;
    theta1 = -alfa;

end

== stateflow chart quadrupedRobot/controller/原地机身YAW角变化演示（有误）/此处可以添加到Kinematics中 ==
  state off
    X_RF1 = X_RF;
    Y_RF1 = Y_RF;
    Z_RF1 = Z_RF;
    X_RR1=X_RR;
    Y_RR1 = Y_RR;
    Z_RR1 = Z_RR;
    X_LF1 =X_LF;
    Y_LF1 =Y_LF;
    Z_LF1 = Z_LF;
    X_LR1 = X_LR;
    Y_LR1 = Y_LR
    Z_LR1 = Z_LR;
  state on
    X_RF1 = X_S;
    Y_RF1 = Y_S;
    Z_RF1 = Z_S;
    X_RR1 = X_S;
    Y_RR1 = Y_S;
    Z_RR1 = Z_S;
    X_LF1 = X_S;
    Y_LF1 = Y_S;
    Z_LF1 = Z_S;
    X_LR1 = X_S;
    Y_LR1 = Y_S;
    Z_LR1 = Z_S;
  (default) -> on
  off -> on : [t<=0.3]
  on -> off : [t>0.3]
  data: t input; X_S input; Y_S input; Z_S input; X_RF input; Y_RF input; Z_RF input; X_RR input; Z_RR input; Y_RR input; Y_LF input; Z_LF input; X_LF input; X_LR input; Z_LR input; Y_LR input; Z_LR1 output; X_LR1 output; X_LF1 output; Z_LF1 output; Y_LF1 output; Y_RR1 output; Z_RR1 output; X_RR1 output; Z_RF1 output; Y_RF1 output; X_RF1 output; Y_LR1 output

== matlab function quadrupedRobot/controller/原地机身YAW角变化演示（有误）/MATLAB Function ==
  data: x0foot input; y0foot input; yaw input; XY_RF output; XY_RR output; XY_LF output; XY_LR output; BodyWidth parameter; BodyCenter_To_Arm parameter
function [XY_RF,XY_RR,XY_LF,XY_LR] = YawXYZgenerator(x0foot,y0foot,yaw, BodyWidth, BodyCenter_To_Arm)%最初y
   
    L0 = BodyCenter_To_Arm;
    L = sqrt ( (BodyWidth/2)^2 + L0^2) ;
    theta1 = atand(BodyWidth/L0)+yaw;
    armVector0= [- x0foot,-y0foot]';
    armMovingVector = [L*cosd(theta1)-L0,L*sind(theta1)-BodyWidth/2]';
    TransMatrix = Axis0_To_Axis1(yaw);
    
    %RF的XY
    armVector0prejection = TransMatrix*armVector0;
    armMovingVector0prejection = TransMatrix*armMovingVector;
    XY_RF = [armVector0prejection(1)+armMovingVector0prejection(1),...
             armVector0prejection(2)+armMovingVector0prejection(2) ];
    XY_RF = -XY_RF;%求得的向量方向不对，故加负号
    
    
    %LF
    XY_LF = [armVector0prejection(1)-armMovingVector0prejection(1),...
             armVector0prejection(2)-armMovingVector0prejection(2) ];
    XY_LF = -XY_LF;%求得的向量方向不对，故加负号
    
   %LR
   XY_LR = [-XY_RF(1),XY_RF(2)];
   
   %RR
   XY_RR = [-XY_LF(1),XY_LF(2)];
end



  
function TransMatrix = Axis0_To_Axis1(yaw)%yaw为偏航角
    TransMatrix = [
                    cosd(yaw) sind(yaw);...
                    -sind(yaw) cosd(yaw);...
                  ];




end

== matlab function quadrupedRobot/controller/原地机身ROLL PITCH YAW三角变化演示（正确）/Kinematics ==
  data: POrAngle_RF output; XYZ input; POrAngle_RR output; POrAngle_LF output; POrAngle_LR output; L1 parameter; L2 parameter; L3 parameter; Mark parameter
function [POrAngle_RF,POrAngle_RR,POrAngle_LF,POrAngle_LR] = fcn(XYZ, L1, L2, L3, Mark)%L1 L2 L3 MARK是内置数值
    



%     RF_XYZ = XYZ(1:3);%右前腿坐标
%     RR_XYZ = XYZ(4:6);
%     LF_XYZ = XYZ(7:9);
%     LR_XYZ = XYZ(10:12);
    
   POrAngle_RF = zeros(1,3);
   POrAngle_RR = zeros(1,3);
   POrAngle_LF = zeros(1,3);
   POrAngle_LR = zeros(1,3);
%     POrAngle1=0;
%     POrAngle2=0;
%     POrAngle3=0;
    Theta_Total = zeros(4,3);%用以装载角度
    XYZ_Total   = zeros(4,3);%用以装载XYZ
    switch Mark
        case 1 %计算逆运动学
           for K=1:4  %依次算四条腿的逆解
                [POrAngle1,POrAngle2,POrAngle3]=inverseKinematics(L1,L2,L3,XYZ(3*K-2),XYZ(3*K-1),XYZ(3*K));
                Theta_Total(K,1) = POrAngle1;
                Theta_Total(K,2) = POrAngle2;
                Theta_Total(K,3) = POrAngle3;
           end
           POrAngle_RF = Theta_Total(1,:) ;
           POrAngle_RR = Theta_Total(2,:) ;
           POrAngle_LF = Theta_Total(3,:) ;
           POrAngle_LR = Theta_Total(4,:) ;
        case 0 
            for K=1:4  %依次算四条腿的逆解
                [POrAngle1,POrAngle2,POrAngle3]=forwardKinematics(L1,L2,L3,XYZ(3*K-2),XYZ(3*K-1),XYZ(3*K));
                XYZ_Total(K,1) = POrAngle1;
                XYZ_Total(K,2) = POrAngle2;
                XYZ_Total(K,3) = POrAngle3;
           end
           POrAngle_RF = XYZ_Total(1,:) ;
           POrAngle_RR = XYZ_Total(2,:) ;
           POrAngle_LF = XYZ_Total(3,:) ;
           POrAngle_LR = XYZ_Total(4,:) ;
    end
    
    
    
    
    
    
    
    
   
    
end



function [x,y,z]=forwardKinematics(a,L1,L2,theta0,theta1,theta2)
    
    H = L1*cosd(theta1)+L2*cosd(theta1+theta2);
    x = L1*sind(theta1)+L2*sind(theta1+theta2);
    z = -H*cosd(theta0)+a*sind(theta0);
    y = a*cosd(theta0)+H*sind(theta0);
end

function [theta0,theta1,theta2]=inverseKinematics(a,L1,L2,x,y,z)

    h = a;
    hu = L1;
    hl = L2;
    %
    y = -y;
    z = -(abs(z));
    dyz = sqrt(y^2+z^2);
    lyz = sqrt(dyz^2-a^2);
    gamma_yz = -atand(y/z);
    gamma_h_offset = -atand(h/lyz);
    gamma = gamma_yz-gamma_h_offset;
    theta0 = -gamma;
    %
    lxzp =  sqrt(lyz^2+x^2);
    n = (lxzp^2-hl^2-hu^2)/2/hu;
    beta = -acosd(n/hl);
    theta2 = -beta ;
    %
    alfa_xzp = -atand(x/lyz);
    alfa_off = acosd((hu+n)/lxzp);
    alfa = alfa_xzp+alfa_off;
    theta1 = -alfa;

end

== matlab function quadrupedRobot/controller/原地机身ROLL PITCH YAW三角变化演示（正确）/YAW 角发生器 ==
  data: x0foot input; y0foot input; yaw input; XY_RF output; XY_RR output; XY_LF output; XY_LR output; BodyWidth parameter; BodyCenter_To_Arm parameter
function [XY_RF,XY_RR,XY_LF,XY_LR] = YawXYZgenerator(x0foot,y0foot,yaw, BodyWidth, BodyCenter_To_Arm)%最初y
   
    L0 = BodyCenter_To_Arm;
    L = sqrt ( (BodyWidth/2)^2 + L0^2) ;
    theta1 = atand(BodyWidth/L0/2)+yaw;
    armVector0= [- x0foot,-y0foot]';
    armMovingVector = [L*cosd(theta1)-L0,L*sind(theta1)-BodyWidth/2]';
    TransMatrix = Axis0_To_Axis1(yaw);
    
    %RF的XY
    armVector0prejection = TransMatrix*armVector0;
    armMovingVector0prejection = TransMatrix*armMovingVector;
    XY_RF = [armVector0prejection(1)+armMovingVector0prejection(1),...
             armVector0prejection(2)+armMovingVector0prejection(2) ];
    XY_RF = -XY_RF;%求得的向量方向不对，故加负号
    
    if yaw~=0
        %LF
        XY_LF = [armVector0prejection(1)-armMovingVector0prejection(1),...
                 armVector0prejection(2)-armMovingVector0prejection(2) ];
        XY_LF = -XY_LF;%求得的向量方向不对，故加负号

       %LR
       XY_LR = [-XY_RF(1),XY_RF(2)];
%         XY_LR = [armVector0prejection(1)-armMovingVector0prejection(1),...
%                  armVector0prejection(2)-armMovingVector0prejection(2) ];
%         XY_LR = -XY_LR;%求得的向量方向不对，故加负号
       %RR
%         XY_RR = [armVector0prejection(1)-armMovingVector0prejection(1),...
%                  armVector0prejection(2)-armMovingVector0prejection(2) ];
%         XY_RR = -XY_LR;%求得的向量方向不对，故加负号       
        XY_RR = [-XY_LF(1),XY_LF(2)];
    else
        XY_LF = XY_RF;
        XY_LR = XY_RF;
        XY_RR = XY_RF;
    end
    
end



  
function TransMatrix = Axis0_To_Axis1(yaw)%yaw为偏航角
    TransMatrix = [
                    cosd(yaw) sind(yaw);...
                    -sind(yaw) cosd(yaw);...
                  ];




end

== stateflow chart quadrupedRobot/controller/原地机身ROLL PITCH YAW三角变化演示（正确）/此处可以添加到Kinematics中 ==
  state off
    X_RF1 = X_RF;
    Y_RF1 = Y_RF;
    Z_RF1 = Z_RF;
    X_RR1=X_RR;
    Y_RR1 = Y_RR;
    Z_RR1 = Z_RR;
    X_LF1 =X_LF;
    Y_LF1 =Y_LF;
    Z_LF1 = Z_LF;
    X_LR1 = X_LR;
    Y_LR1 = Y_LR
    Z_LR1 = Z_LR;
  state on
    X_RF1 = X_S;
    Y_RF1 = Y_S;
    Z_RF1 = Z_S;
    X_RR1 = X_S;
    Y_RR1 = Y_S;
    Z_RR1 = Z_S;
    X_LF1 = X_S;
    Y_LF1 = Y_S;
    Z_LF1 = Z_S;
    X_LR1 = X_S;
    Y_LR1 = Y_S;
    Z_LR1 = Z_S;
  (default) -> on
  off -> on : [t<=0.5]
  on -> off : [t>0.5]
  data: t input; X_S input; Y_S input; Z_S input; X_RF input; Y_RF input; Z_RF input; X_RR input; Z_RR input; Y_RR input; Y_LF input; Z_LF input; X_LF input; X_LR input; Z_LR input; Y_LR input; Z_LR1 output; X_LR1 output; X_LF1 output; Z_LF1 output; Y_LF1 output; Y_RR1 output; Z_RR1 output; X_RR1 output; Z_RF1 output; Y_RF1 output; X_RF1 output; Y_LR1 output

== matlab function quadrupedRobot/controller/原地机身ROLL PITCH YAW三角变化演示（正确）/ROLL发生器 以右前腿高度不变为参考 ==
  data: rollAngle input; y1 input; y2 input; Z2 input; Z1 output; Z2 output; BodyWidth parameter
function [Z1,Z2] = fcn(rollAngle, y1,y2,Z2,BodyWidth)

% rollAngle = u(1) ;
% y1        = u(2) ;
% y2        = u(3) ;
% Z2        = u(4) ;   %参考高度

[Z1]=roll_angle_2_Z(rollAngle,BodyWidth,y1,y2,Z2);


end

function [Z1]=roll_angle_2_Z(rollAngle,BodyWidth,y1,y2,Z2) %单位度
    %y1是右边的
    %y2是左边的 其大小参考肩部坐标系
    
    deltaZ = tand(rollAngle)*(BodyWidth+(y1+y2));
    Z1 = Z2 + deltaZ;

end

== matlab function quadrupedRobot/controller/原地机身ROLL PITCH YAW三角变化演示（正确）/PITCH发生器 ==
  data: pitchAngle input; x1 input; x2 input; Z2 input; Z1 output; Z2 output; BodyCenter_To_Arm parameter
function [Z1,Z2] = fcn(pitchAngle,x1,x2,Z2, BodyCenter_To_Arm)

% pitchAngle = u(1) ;
% x1        = u(3) ;
% x2        = u(4) ;
% Z2        = u(5) ;   %参考高度

[Z1]=roll_angle_2_Z(pitchAngle,BodyCenter_To_Arm,x1,x2,Z2);


end

function [Z1]=roll_angle_2_Z(rollAngle,BodyCenter_To_Arm,x1,x2,Z2) %单位度
    %y1是右边的
    %y2是左边的 其大小参考肩部坐标系
    
    deltaZ = tand(rollAngle)*(BodyCenter_To_Arm*2+abs(x1-x2));
    Z1 = Z2 + deltaZ;

end

== matlab function quadrupedRobot/controller/原地机身ROLL角变化演示/theta2height ==
  data: u input; Z1 output; Z2 output
function [Z1,Z2] = fcn(u)

rollAngle = u(1) ;
BodyWidth = u(2) ;
y1        = u(3) ;
y2        = u(4) ;
Z2        = u(5) ;   %参考高度

[Z1]=roll_angle_2_Z(rollAngle,BodyWidth,y1,y2,Z2);


end

function [Z1]=roll_angle_2_Z(rollAngle,BodyWidth,y1,y2,Z2) %单位度
    %y1是右边的
    %y2是左边的 其大小参考肩部坐标系
    
    deltaZ = tand(rollAngle)*(BodyWidth+y1+y2);
    Z1 = Z2 + deltaZ;

end

== stateflow chart quadrupedRobot/controller/对角步态演示/此处可以添加到Kinematics中 ==
  state off
    X_RF1 = X_RF;
    Y_RF1 = Y_RF;
    Z_RF1 = Z_RF;
    X_RR1=X_RR;
    Y_RR1 = Y_RR;
    Z_RR1 = Z_RR;
    X_LF1 =X_LF;
    Y_LF1 =Y_LF;
    Z_LF1 = Z_LF;
    X_LR1 = X_LR;
    Y_LR1 = Y_LR
    Z_LR1 = Z_LR;
  state on
    X_RF1 = X_S;
    Y_RF1 = Y_S;
    Z_RF1 = Z_S;
    X_RR1 = X_S;
    Y_RR1 = Y_S;
    Z_RR1 = Z_S;
    X_LF1 = X_S;
    Y_LF1 = Y_S;
    Z_LF1 = Z_S;
    X_LR1 = X_S;
    Y_LR1 = Y_S;
    Z_LR1 = Z_S;
  (default) -> on
  off -> on : [t<=0.3]
  on -> off : [t>0.3]
  data: t input; X_S input; Y_S input; Z_S input; X_RF input; Y_RF input; Z_RF input; X_RR input; Z_RR input; Y_RR input; Y_LF input; Z_LF input; X_LF input; X_LR input; Z_LR input; Y_LR input; Z_LR1 output; X_LR1 output; X_LF1 output; Z_LF1 output; Y_LF1 output; Y_RR1 output; Z_RR1 output; X_RR1 output; Z_RF1 output; Y_RF1 output; X_RF1 output; Y_LR1 output

== matlab function quadrupedRobot/controller/对角步态演示/Kinematics3 ==
  data: POrAngle_RF output; XYZ input; POrAngle_RR output; POrAngle_LF output; POrAngle_LR output; L1 parameter; L2 parameter; L3 parameter; Mark parameter
function [POrAngle_RF,POrAngle_RR,POrAngle_LF,POrAngle_LR] = fcn(XYZ, L1, L2, L3, Mark)%L1 L2 L3 MARK是内置数值
    



%     RF_XYZ = XYZ(1:3);%右前腿坐标
%     RR_XYZ = XYZ(4:6);
%     LF_XYZ = XYZ(7:9);
%     LR_XYZ = XYZ(10:12);
    
   POrAngle_RF = zeros(1,3);
   POrAngle_RR = zeros(1,3);
   POrAngle_LF = zeros(1,3);
   POrAngle_LR = zeros(1,3);
%     POrAngle1=0;
%     POrAngle2=0;
%     POrAngle3=0;
    Theta_Total = zeros(4,3);%用以装载角度
    XYZ_Total   = zeros(4,3);%用以装载XYZ
    switch Mark
        case 1 %计算逆运动学
           for K=1:4  %依次算四条腿的逆解
                [POrAngle1,POrAngle2,POrAngle3]=inverseKinematics(L1,L2,L3,XYZ(3*K-2),XYZ(3*K-1),XYZ(3*K));
                Theta_Total(K,1) = POrAngle1;
                Theta_Total(K,2) = POrAngle2;
                Theta_Total(K,3) = POrAngle3;
           end
           POrAngle_RF = Theta_Total(1,:) ;
           POrAngle_RR = Theta_Total(2,:) ;
           POrAngle_LF = Theta_Total(3,:) ;
           POrAngle_LR = Theta_Total(4,:) ;
        case 0 
            for K=1:4  %依次算四条腿的逆解
                [POrAngle1,POrAngle2,POrAngle3]=forwardKinematics(L1,L2,L3,XYZ(3*K-2),XYZ(3*K-1),XYZ(3*K));
                XYZ_Total(K,1) = POrAngle1;
                XYZ_Total(K,2) = POrAngle2;
                XYZ_Total(K,3) = POrAngle3;
           end
           POrAngle_RF = XYZ_Total(1,:) ;
           POrAngle_RR = XYZ_Total(2,:) ;
           POrAngle_LF = XYZ_Total(3,:) ;
           POrAngle_LR = XYZ_Total(4,:) ;
    end
    
    
    
    
    
    
    
    
   
    
end



function [x,y,z]=forwardKinematics(a,L1,L2,theta0,theta1,theta2)
    
    H = L1*cosd(theta1)+L2*cosd(theta1+theta2);
    x = L1*sind(theta1)+L2*sind(theta1+theta2);
    z = -H*cosd(theta0)+a*sind(theta0);
    y = a*cosd(theta0)+H*sind(theta0);
end

function [theta0,theta1,theta2]=inverseKinematics(a,L1,L2,x,y,z)

    h = a;
    hu = L1;
    hl = L2;
    %
    y = -y;
    z = -(abs(z));
    dyz = sqrt(y^2+z^2);
    lyz = sqrt(dyz^2-a^2);
    gamma_yz = -atand(y/z);
    gamma_h_offset = -atand(h/lyz);
    gamma = gamma_yz-gamma_h_offset;
    theta0 = -gamma;
    %
    lxzp =  sqrt(lyz^2+x^2);
    n = (lxzp^2-hl^2-hu^2)/2/hu;
    beta = -acosd(n/hl);
    theta2 = -beta ;
    %
    alfa_xzp = -atand(x/lyz);
    alfa_off = acosd((hu+n)/lxzp);
    alfa = alfa_xzp+alfa_off;
    theta1 = -alfa;

end

== stateflow chart quadrupedRobot/controller/原地机身ROLL角变化演示/延时等待躯体稳定 ==
  state off
    X_RF1 = X_RF;
    Y_RF1 = Y_RF;
    Z_RF1 = Z_RF;
    X_RR1=X_RR;
    Y_RR1 = Y_RR;
    Z_RR1 = Z_RR;
    X_LF1 =X_LF;
    Y_LF1 =Y_LF;
    Z_LF1 = Z_LF;
    X_LR1 = X_LR;
    Y_LR1 = Y_LR
    Z_LR1 = Z_LR;
  state on
    X_RF1 = X_S;
    Y_RF1 = Y_S;
    Z_RF1 = Z_S;
    X_RR1 = X_S;
    Y_RR1 = Y_S;
    Z_RR1 = Z_S;
    X_LF1 = X_S;
    Y_LF1 = Y_S;
    Z_LF1 = Z_S;
    X_LR1 = X_S;
    Y_LR1 = Y_S;
    Z_LR1 = Z_S;
  (default) -> on
  off -> on : [t<=0.8]
  on -> off : [t>0.8]
  data: t input; X_S input; Y_S input; Z_S input; X_RF input; Y_RF input; Z_RF input; X_RR input; Z_RR input; Y_RR input; Y_LF input; Z_LF input; X_LF input; X_LR input; Z_LR input; Y_LR input; Z_LR1 output; X_LR1 output; X_LF1 output; Z_LF1 output; Y_LF1 output; Y_RR1 output; Z_RR1 output; X_RR1 output; Z_RF1 output; Y_RF1 output; X_RF1 output; Y_LR1 output
